simulink model "Closed_loop_PID_nterferometer"  (R2019b)
settings: Solver=ode3  StartTime=0.0  StopTime=0.5  FixedStep=0.00001  RelTol=1e-3  EnableMultiTasking=on
InitFcn:
  | A =1
  | V =1
libraries: simulink x2, dsparch4 x1
settings Model: Creator=Roberta Martin  LastModifiedBy=Stinky
settings DataIOCC: LimitDataPoints=on  SaveFormat=Array  ReturnWorkspaceOutputs=off
settings OptimizationCC: LifeSpan=inf
settings DebuggingCC: UnderspecifiedInitializationDetection=Classic  MergeDetectMultiDrivingBlocksExec=none  SolverPrmCheckMsg=warning  AllowSymbolicDim=off  SFUnexpectedBacktrackingDiag=warning  SFNoUnconditionalDefaultTransitionDiag=warning  SFExecutionAtInitializationDiag=none  ArithmeticOperatorsInVariantConditions=warning
settings HardwareCC: ProdBitPerPointer=32  ProdBitPerSizeT=32  ProdBitPerPtrDiffT=32  ProdLargestAtomicFloat=None  ProdIntDivRoundTo=Undefined  ProdEndianess=Unspecified  ProdWordSize=32  ProdHWDeviceType=32-bit Generic
settings ModelReferenceCC: PropagateSignalLabelsOutOfModel=off
settings SFSimCC: SimUseLocalCustomCode=off  CustomCodeUndefinedFunction=UseInterfaceOnly
settings RTWCC: RTWUseLocalCustomCode=off
settings CodeAppCC: StateflowObjectComments=on
settings GRTTargetCC: TargetLangStandard=C89/C90 (ANSI)  GeneratePreprocessorConditionals=Disable all
settings ConfigComp: CovMetricSettings=dw  CovHtmlReporting=on  CovSaveCumulativeToWorkspaceVar=on  CovSaveSingleToWorkspaceVar=on  CovExternalEMLEnable=off
settings SimscapeCC: SimscapeNormalizeSystem=off

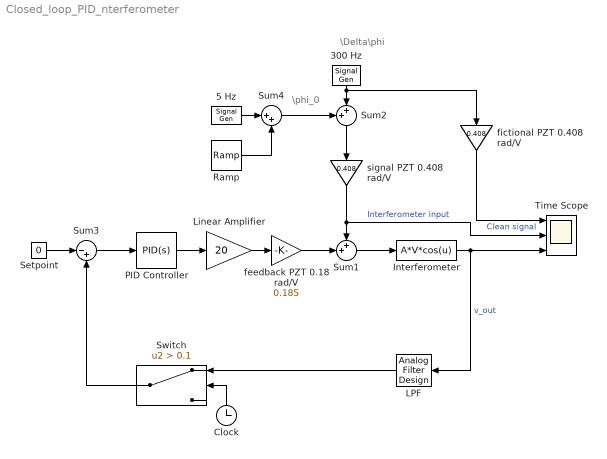
== system Closed_loop_PID_nterferometer ==
  note: \phi_0
  note: \Delta\phi
  " 5 Hz" : SignalGenerator  Amplitude=2  Frequency=5
  "300 Hz " : SignalGenerator  Frequency=300
  Clock : Clock
  Interferometer : Fcn  Expr=A*V*cos(u)
  LPF : dsparch4/Analog Filter Design  method=Butterworth  filttype=Lowpass  N=1  Wlo=20*2*pi()  Whi=80  Rp=2  Rs=40
  Linear Amplifier : Gain  Gain=20
  PID Controller : simulink/Continuous/PID Controller  Controller=PID  Form=Parallel  TimeDomain=Continuous-time  SampleTime=-1  IntegratorMethod=Forward Euler  FilterMethod=Forward Euler  ControllerParametersSource=internal  P=136  I=1  D=0  UseFilter=on  N=0  TunerSelectOption=Transfer Function Based (PID Tuner App)  InitialConditionSource=internal  InitialConditionForIntegrator=0  InitialConditionForFilter=0  DifferentiatorICPrevScaledInput=0  ExternalReset=none  TrackingMode=off  Kt=1  LimitOutput=off  UpperSaturationLimit=inf  LowerSaturationLimit=-inf  LinearizeAsGain=on  AntiWindupMode=none  Kb=1  POutMin=[]  POutMax=[]  IOutMin=[]  IOutMax=[]  DOutMin=[]  DOutMax=[]  NOutMin=[]  NOutMax=[]  SumOutMin=[]  SumOutMax=[]  SaturationOutMin=[]  SaturationOutMax=[]  PParamMin=[]  PParamMax=[]  IParamMin=[]  IParamMax=[]  DParamMin=[]  DParamMax=[]  NParamMin=[]  NParamMax=[]  KbParamMin=[]  KbParamMax=[]  KtParamMin=[]  KtParamMax=[]  KbOutMin=[]  KbOutMax=[]  KtOutMin=[]  KtOutMax=[]  IntegratorOutMin=[]  IntegratorOutMax=[]  FilterOutMin=[]  FilterOutMax=[]  SumI1OutMin=[]  SumI1OutMax=[]  SumI2OutMin=[]  SumI2OutMax=[]  SumI3OutMin=[]  SumI3OutMax=[]  SumI4OutMin=[]  SumI4OutMax=[]  SumDOutMin=[]  SumDOutMax=[]  DifferentiatorOutMin=[]  DifferentiatorOutMax=[]  FilterDiffOutCoefMin=[]  FilterDiffOutCoefMax=[]  ReciprocalOutMin=[]  ReciprocalOutMax=[]  SumDenOutMin=[]  SumDenOutMax=[]  SumNumOutMin=[]  SumNumOutMax=[]  DivideOutMin=[]  DivideOutMax=[]  IntegratorContinuousStateAttributes=''  IntegratorStateMustResolveToSignalObject=off  IntegratorRTWStateStorageClass=Auto  FilterContinuousStateAttributes=''  FilterStateMustResolveToSignalObject=off  FilterRTWStateStorageClass=Auto  ParallelPVariant=InternalParameters  IdealPVariant=Disabled  IVariant=InternalParameters  DVariant=InternalParameters  IntegratorVariant=Continuous  SatVariant=Disabled  AWVariant=Passthrough  PCopyVariant=Disabled  TRVariant=Disabled  FdbkBlocksVariant=Forward  IdealPFdbkVariant=Disabled  SatFdbkVariant=Disabled  DerivativeFilterVariant=ContFilter  NVariant=InternalParameters  NCopyVariant=Disabled  FilterICVariant=InternalICsFilter  IntegratorICVariant=InternalICs  ExternalResetVariant=Disabled  TRSumVariant=Passthrough  SumFdbkVariant=Disabled  SumVariant=Sum_PID
  Ramp : simulink/Sources/Ramp  slope=50  start=0  InitialOutput=0
  Setpoint : Constant  Value=0
  Sum1 : Sum  Inputs=++|
  Sum2 : Sum  Inputs=++|
  Sum3 : Sum  Inputs=|-+
  Sum4 : Sum  Inputs=|++
  Switch : Switch  Criteria=u2 > Threshold  Threshold=0.1
  Time Scope : Scope  NumInputPorts=3
  feedback PZT 0.18 rad/V : Gain  Gain=0.185
  fictional PZT 0.408 rad/V : Gain  Gain=0.408
  signal PZT 0.408 rad/V : Gain  Gain=0.408
  wires:
  Interferometer/1 -> LPF/1, Time Scope/3  "v_out"
  Sum1/1 -> Interferometer/1
  signal PZT 0.408 rad/V/1 -> Time Scope/2, Sum1/1  "Interferometer input"
  Sum2/1 -> signal PZT 0.408 rad/V/1
  "300 Hz "/1 -> Sum2/2, fictional PZT 0.408 rad/V/1
  Setpoint/1 -> Sum3/1
  fictional PZT 0.408 rad/V/1 -> Time Scope/1  "Clean signal"
  Switch/1 -> Sum3/2
  Clock/1 -> Switch/2
  Sum4/1 -> Sum2/1
  " 5 Hz"/1 -> Sum4/1
  Ramp/1 -> Sum4/2
  Sum3/1 -> PID Controller/1
  LPF/1 -> Switch/1
  Linear Amplifier/1 -> feedback PZT 0.18 rad/V/1
  feedback PZT 0.18 rad/V/1 -> Sum1/2
  PID Controller/1 -> Linear Amplifier/1
